simulink model "das2test"  (R2019b)
settings: Solver=ode4  StartTime=0.0  StopTime=10  FixedStep=Auto  RelTol=1e-3  EnableMultiTasking=on
libraries: simulink x1
settings Model: ParamWorkspaceSource=ReferencedWorkspace  ExtModeAutoUpdateStatusClock=off  Creator=chadwick  LastModifiedBy=clamack
settings DataIOCC: LimitDataPoints=on  MaxDataPoints=20000  SaveFinalState=on  SaveFormat=Array  SignalLoggingSaveFormat=ModelDataLogs  SaveOutput=off  SignalLogging=off  SaveTime=off  ReturnWorkspaceOutputs=off
settings OptimizationCC: BlockReduction=off  DefaultParameterBehavior=Inlined  OptimizeBlockIOStorage=off  BufferReuse=off  GlobalBufferReuse=off  ExpressionFolding=off  ExpressionDepthLimit=2147483647  LocalBlockOutputs=off  InitFltsAndDblsToZero=on  LifeSpan=inf  OptimizeDataStoreBuffers=off  BusAssignmentInplaceUpdate=off
settings DebuggingCC: SaveWithParameterizedLinksMsg=none  UnderspecifiedInitializationDetection=Classic  MergeDetectMultiDrivingBlocksExec=none  SignalResolutionControl=TryResolveAllWithWarning  SolverPrmCheckMsg=warning  MultiTaskDSMMsg=warning  MultiTaskCondExecSysMsg=none  FcnCallInpInsideContextMsg=warning  StateNameClashWarn=warning  SFUnexpectedBacktrackingDiag=warning  SFNoUnconditionalDefaultTransitionDiag=warning  SFExecutionAtInitializationDiag=none  ArithmeticOperatorsInVariantConditions=warning
settings HardwareCC: ProdBitPerPointer=32  ProdBitPerSizeT=32  ProdBitPerPtrDiffT=32  ProdLargestAtomicFloat=None  ProdWordSize=32  ProdHWDeviceType=32-bit xPC Target (Intel Pentium)
settings ModelReferenceCC: ModelReferenceNumInstancesAllowed=Single  PropagateSignalLabelsOutOfModel=off
settings SFSimCC: SimParseCustomCode=off
settings RTWCC: Description=xPC Target  SystemTargetFile=xpctarget.tlc  TemplateMakefile=xpc_default_tmf  CustomInclude=..\..\..\tools\sdbio\trunk\ ..\..\..\das2\model\trunk\ ..\..\..\das2\das2sim\trunk\  CustomSource=sdbio.c sdlib.c model_d.c
settings CodeAppCC: StateflowObjectComments=on
settings TargetCC: TargetFcnLib=ansi_tfl_tmw.mat  CompOptLevelCompliant=off  GeneratePreprocessorConditionals=Use local settings  MatFileLogging=on  PreserveStateflowLocalDataDimensions=off
settings ConfigComp: CovMetricSettings=dw  CovHtmlReporting=on  CovSaveCumulativeToWorkspaceVar=on  CovSaveSingleToWorkspaceVar=on

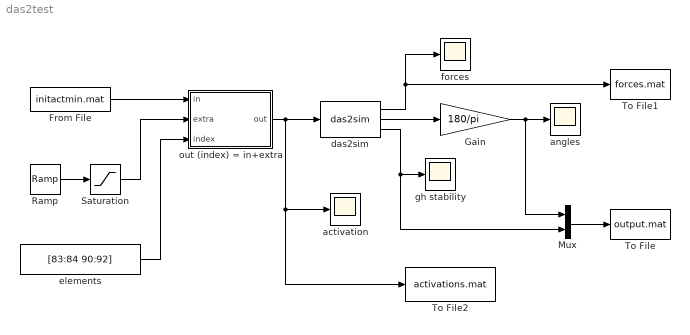
== system das2test ==
  From File : FromFile  FileName=initactmin.mat  SampleTime=0.001
  Gain : Gain  Gain=180/pi
  Mux : Mux  Inputs=2
  Ramp : simulink/Sources/Ramp  slope=0.2  start=1  InitialOutput=0
  Saturation : Saturate  UpperLimit=1  LowerLimit=0
  To File : ToFile  Filename=output.mat  MatrixName=output
      settings: Decimation=10
  To File1 : ToFile  Filename=forces.mat  MatrixName=forces
      settings: Decimation=10
  To File2 : ToFile  Filename=activations.mat  MatrixName=act
      settings: Decimation=20
  activation : Scope
  angles : Scope
  das2sim : S-Function  FunctionName=das2sim  SFunctionDeploymentMode=off  EnableBusSupport=off
  elements : Constant  Value=[83:84 90:92]
  forces : Scope
  gh stability : Scope
  out (index) = in+extra : MATLAB Function  TreatAsAtomicUnit=on
  wires:
  das2sim/2 -> Gain/1
  Gain/1 -> angles/1, Mux/1
  das2sim/3 -> gh stability/1, Mux/2
  out (index) = in+extra/1(out) -> das2sim/1, activation/1, To File2/1
  Mux/1 -> To File/1
  das2sim/1 -> forces/1, To File1/1
  From File/1 -> out (index) = in+extra/1(in)
  Ramp/1 -> Saturation/1
  elements/1 -> out (index) = in+extra/3(index)
  Saturation/1 -> out (index) = in+extra/2(extra)

== matlab function das2test/out (index) = in+extra ==
  data: in input; out output; extra input; index input
function out = inject(in,extra,index)
% adds an EXTRA signal to specified elements (INDEX) of the IN vector

out = in;
for i=index
    out(i)=in(i)+extra;
end
